simulink library "lib_Convection_HeatCapIdealGas"  (R2015a)
settings: Solver=ode45  StartTime=0.0  StopTime=10.0  RelTol=1e-3
settings Model: Creator=jlkratz  LastModifiedBy=jlkratz

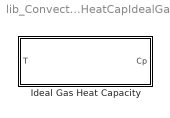
== system lib_Convection_HeatCapIdealGas ==
  Ideal Gas Heat Capacity : Subsystem  mask(TSAT: Ideal Gas Heat Capacity){a_M=28.11, b_M=0.1967*10^-2, c_M=0.4802*10^-5, d_M=1.966*10^-9}
      mask prompts: a_M "a_M - Coefficient 1"; b_M "b_M - Coefficient 2"; c_M "c_M - Coefficient 3"; d_M "d_M - Coefficient 4"
      mask help:
      | This block uses a cubic fitted correlation:
      |
      | Cp = a + b*T + c*T^2 + d*T^3
      |
      | to approximate the heat capacity of an ideal gas. The coefficients a, b, c, and d will depend on the gas and the temperature range which the correlation is valid may differ as well. The user is cautioned to observe the limitations of the correlation.
      |
      | Some values of the coefficients for common gases can be found in the help menu of this block.
      mask Help: web(which('Convection_TSAT_HeatCapIdealGas.html'),'-helpbrowser')

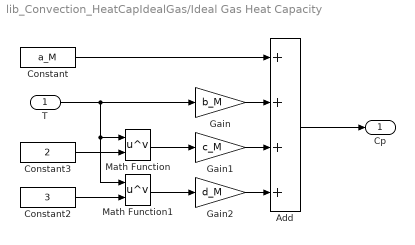
== system lib_Convection_HeatCapIdealGas/Ideal Gas Heat Capacity ==
  T : Inport
  Add : Sum  Inputs=++++
  Constant : Constant  Value=a_M
  Constant2 : Constant  Value=3
  Constant3 : Constant  Value=2
  Gain : Gain  Gain=b_M
  Gain1 : Gain  Gain=c_M
  Gain2 : Gain  Gain=d_M
  Math Function : Math  Operator=pow  SaturateOnIntegerOverflow=on
  Math Function1 : Math  Operator=pow  SaturateOnIntegerOverflow=on
  Cp : Outport
  wires:
  Add/1 -> Cp/1
  Math Function1/1 -> Gain2/1
  Math Function/1 -> Gain1/1
  T/1 -> Gain/1, Math Function/1, Math Function1/1
  Constant3/1 -> Math Function/2
  Constant/1 -> Add/1
  Gain/1 -> Add/2
  Gain2/1 -> Add/4
  Constant2/1 -> Math Function1/2
  Gain1/1 -> Add/3
